simulink model "SF051A_SnsrOffsLrng"  (R2013b)
settings: Solver=FixedStepDiscrete  SolverMode=SingleTasking  StartTime=0.0  StopTime=1  FixedStep=0.002  RelTol=1e-3
values from neighbouring files (symbols this model uses):
  ARCHGLBPRM_10MILLISEC_SEC_F32 = DataDict.Constant    [SF051A_SnsrOffsLrng_DataDict.m]
  ARCHGLBPRM_2MILLISEC_SEC_F32 = DataDict.Constant    [SF051A_SnsrOffsLrng_DataDict.m]
  ARCHGLBPRM_2PI_ULS_F32 = DataDict.Constant    [SF051A_SnsrOffsLrng_DataDict.m]
  ARCHGLBPRM_FLOATZEROTHD_ULS_F32 = DataDict.Constant    [SF051A_SnsrOffsLrng_DataDict.m]
  ARCHGLBPRM_PIOVER180_ULS_F32 = DataDict.Constant    [SF051A_SnsrOffsLrng_DataDict.m]
  CNV100MICROSECTOSEC_SECPERCNT_F32 = DataDict.Constant    [SF051A_SnsrOffsLrng_DataDict.m]
  COVRAMTRXNIT_ULS_F32 = DataDict.Constant    [SF051A_SnsrOffsLrng_DataDict.m]
  HWAGHILIM_HWDEG_F32 = DataDict.Constant    [SF051A_SnsrOffsLrng_DataDict.m]
  HWAUTHYTHD_ULS_F32 = DataDict.Constant    [SF051A_SnsrOffsLrng_DataDict.m]
  HWTQLRNGSTSLRND_CNT_U08 = DataDict.Constant    [SF051A_SnsrOffsLrng_DataDict.m]
  HWTQLRNGSTSNEGOFFS_CNT_U08 = DataDict.Constant    [SF051A_SnsrOffsLrng_DataDict.m]
  HWTQLRNGSTSNOTLRND_CNT_U08 = DataDict.Constant    [SF051A_SnsrOffsLrng_DataDict.m]
  HWTQLRNGSTSPOSOFFS_CNT_U08 = DataDict.Constant    [SF051A_SnsrOffsLrng_DataDict.m]
  HWTQLRNGSTSZEROOFFS_CNT_U08 = DataDict.Constant    [SF051A_SnsrOffsLrng_DataDict.m]
  IDYMTRX_ULS_F32 = DataDict.Constant    [SF051A_SnsrOffsLrng_DataDict.m]
  IVS10MS_ULSPERSEC_F32 = DataDict.Constant    [SF051A_SnsrOffsLrng_DataDict.m]
  LRNGFILTICON_ULS_F32 = DataDict.Constant    [SF051A_SnsrOffsLrng_DataDict.m]
  ONE_ULS_F32 = DataDict.Constant    [SF051A_SnsrOffsLrng_DataDict.m]
  SnsrOffsLrnd = DataDict.NVM    [SF051A_SnsrOffsLrng_DataDict.m]
  SnsrOffsLrngFctEna = DataDict.Calibration    [SF051A_SnsrOffsLrng_DataDict.m]
  SnsrOffsLrngHwAgLrngDrvgDstThd = DataDict.Calibration    [SF051A_SnsrOffsLrng_DataDict.m]
  SnsrOffsLrngHwAgLrngEna = DataDict.Calibration    [SF051A_SnsrOffsLrng_DataDict.m]
  SnsrOffsLrngHwAgLrngHwVelThd = DataDict.Calibration    [SF051A_SnsrOffsLrng_DataDict.m]
  SnsrOffsLrngHwAgLrngSysTqThd = DataDict.Calibration    [SF051A_SnsrOffsLrng_DataDict.m]
  SnsrOffsLrngHwAgLrngSysTqThdMed = DataDict.Calibration    [SF051A_SnsrOffsLrng_DataDict.m]
  SnsrOffsLrngHwAgLrngSysTqThdTrustd = DataDict.Calibration    [SF051A_SnsrOffsLrng_DataDict.m]
  SnsrOffsLrngHwAgLrngSysTqThdWide = DataDict.Calibration    [SF051A_SnsrOffsLrng_DataDict.m]
  SnsrOffsLrngHwAgLrngTi = DataDict.Calibration    [SF051A_SnsrOffsLrng_DataDict.m]
  SnsrOffsLrngHwAgLrngVehSpdThd = DataDict.Calibration    [SF051A_SnsrOffsLrng_DataDict.m]
  SnsrOffsLrngHwAgLrngYawOffsDbnd = DataDict.Calibration    [SF051A_SnsrOffsLrng_DataDict.m]
  SnsrOffsLrngHwAgLrngYawRateThd = DataDict.Calibration    [SF051A_SnsrOffsLrng_DataDict.m]
  SnsrOffsLrngHwAgOffsLim = DataDict.Calibration    [SF051A_SnsrOffsLrng_DataDict.m]
  SnsrOffsLrngHwTqLrngEna = DataDict.Calibration    [SF051A_SnsrOffsLrng_DataDict.m]
  SnsrOffsLrngHwTqLrngEnaTiThd = DataDict.Calibration    [SF051A_SnsrOffsLrng_DataDict.m]
  SnsrOffsLrngHwTqLrngHwAgDbnd = DataDict.Calibration    [SF051A_SnsrOffsLrng_DataDict.m]
  SnsrOffsLrngHwTqLrngHwAgThd = DataDict.Calibration    [SF051A_SnsrOffsLrng_DataDict.m]
  SnsrOffsLrngHwTqLrngHwTqThd = DataDict.Calibration    [SF051A_SnsrOffsLrng_DataDict.m]
  SnsrOffsLrngHwTqLrngHwTqZeroOffsThd = DataDict.Calibration    [SF051A_SnsrOffsLrng_DataDict.m]
  SnsrOffsLrngHwTqLrngHwVelThd = DataDict.Calibration    [SF051A_SnsrOffsLrng_DataDict.m]
  SnsrOffsLrngHwTqLrngMeasTi = DataDict.Calibration    [SF051A_SnsrOffsLrng_DataDict.m]
  SnsrOffsLrngHwTqLrngMeasTiScar = DataDict.Calibration    [SF051A_SnsrOffsLrng_DataDict.m]
  SnsrOffsLrngHwTqLrngSampleImbThd1 = DataDict.Calibration    [SF051A_SnsrOffsLrng_DataDict.m]
  SnsrOffsLrngHwTqLrngSampleImbThd2 = DataDict.Calibration    [SF051A_SnsrOffsLrng_DataDict.m]
  SnsrOffsLrngHwTqLrngSampleThd1 = DataDict.Calibration    [SF051A_SnsrOffsLrng_DataDict.m]
  SnsrOffsLrngHwTqLrngSampleThd2 = DataDict.Calibration    [SF051A_SnsrOffsLrng_DataDict.m]
  SnsrOffsLrngHwTqLrngTiWghtCoeff = DataDict.Calibration    [SF051A_SnsrOffsLrng_DataDict.m]
  SnsrOffsLrngHwTqLrngVehSpdThd = DataDict.Calibration    [SF051A_SnsrOffsLrng_DataDict.m]
  SnsrOffsLrngHwTqOffsLim = DataDict.Calibration    [SF051A_SnsrOffsLrng_DataDict.m]
  SnsrOffsLrngSampleCntForHwTqLrngRst = DataDict.Calibration    [SF051A_SnsrOffsLrng_DataDict.m]
  SnsrOffsLrngTqInpDetnPwrEstimnThd = DataDict.Calibration    [SF051A_SnsrOffsLrng_DataDict.m]
  SnsrOffsLrngTqInpDetnSinGenrAmp = DataDict.Calibration    [SF051A_SnsrOffsLrng_DataDict.m]
  SnsrOffsLrngTqInpDetnSinGenrFrq = DataDict.Calibration    [SF051A_SnsrOffsLrng_DataDict.m]
  SnsrOffsLrngTqInpDetnStg1FilGain = DataDict.Calibration    [SF051A_SnsrOffsLrng_DataDict.m]
  SnsrOffsLrngTqInpDetnStg1WinSize = DataDict.Calibration    [SF051A_SnsrOffsLrng_DataDict.m]
  SnsrOffsLrngTqInpDetnStg2FilGainCen = DataDict.Calibration    [SF051A_SnsrOffsLrng_DataDict.m]
  SnsrOffsLrngTqInpDetnStg2FilGainDwn = DataDict.Calibration    [SF051A_SnsrOffsLrng_DataDict.m]
  SnsrOffsLrngTqInpDetnStg2FilGainUp = DataDict.Calibration    [SF051A_SnsrOffsLrng_DataDict.m]
  SnsrOffsLrngTqInpDetnStg2WinSize = DataDict.Calibration    [SF051A_SnsrOffsLrng_DataDict.m]
  SnsrOffsLrngYawLrngEna = DataDict.Calibration    [SF051A_SnsrOffsLrng_DataDict.m]
  SnsrOffsLrngYawLrngHwAgThd = DataDict.Calibration    [SF051A_SnsrOffsLrng_DataDict.m]
  SnsrOffsLrngYawLrngTi = DataDict.Calibration    [SF051A_SnsrOffsLrng_DataDict.m]
  SnsrOffsLrngYawLrngYawAThd = DataDict.Calibration    [SF051A_SnsrOffsLrng_DataDict.m]
  SnsrOffsLrngYawOffsFrshTiThd = DataDict.Calibration    [SF051A_SnsrOffsLrng_DataDict.m]
  SnsrOffsLrngYawRateOffsLim = DataDict.Calibration    [SF051A_SnsrOffsLrng_DataDict.m]
  SPDCNVN_MTRPERSECPERKPH_F32 = DataDict.Constant    [SF051A_SnsrOffsLrng_DataDict.m]
  SysGlbPrmSysTqRat = DataDict.ImprtdCal    [SF051A_SnsrOffsLrng_DataDict.m]
  TISTEP10MS_MINS_F32 = DataDict.Constant    [SF051A_SnsrOffsLrng_DataDict.m]
  TQINPDETNLOGGAIN_ULS_F32 = DataDict.Constant    [SF051A_SnsrOffsLrng_DataDict.m]
  YAWELPDTIHILIM_MINS_F32 = DataDict.Constant    [SF051A_SnsrOffsLrng_DataDict.m]
  YAWRATENOISE_VEHDEGPERSEC_F32 = DataDict.Constant    [SF051A_SnsrOffsLrng_DataDict.m]
  ZERO_ULS_F32 = DataDict.Constant    [SF051A_SnsrOffsLrng_DataDict.m]
  ZEROVECT_ULS_F32 = DataDict.Constant    [SF051A_SnsrOffsLrng_DataDict.m]
undefined symbols (not defined in the file or in its folder): NvmGetErrSts1
libraries: Fil x34, NxtrLim x20, FixdToFloat x17, FloatToFixd x16, simulink x12, NxtrAbslt x12, NxtrNvM x8, NxtrMath x3
(part 4 of 12)

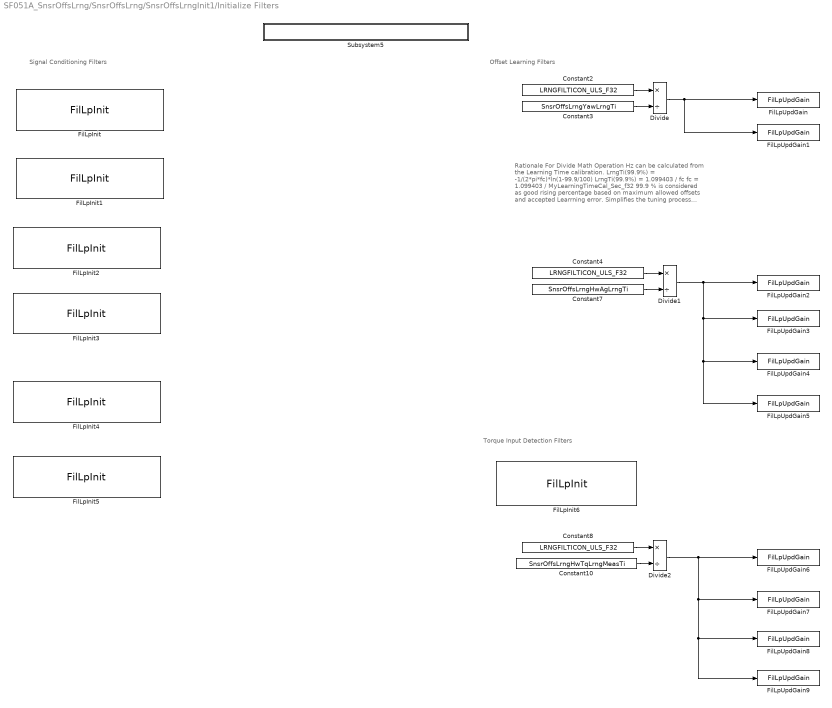
== system SF051A_SnsrOffsLrng/SnsrOffsLrng/SnsrOffsLrngInit1/Initialize Filters ==
  note: Rationale For Divide Math Operation
      |   Hz can be calculated from the Learning Time calibration.
      |   LrngTi(99.9%) = -1/(2*pi*fc)*ln(1-99.9/100)
      |   LrngTi(99.9%) = 1.099403 / fc
      |   fc = 1.099403 / MyLearningTimeCal_Sec_f32
      |
      |   99.9 % is considered as good rising percentage based on
      |   maximum allowed offsets and accepted Learrning error.
      |   Simplifies the tuning process and prevents the customer to
      |   directly find out that we use LPF as the learning method.
  note: Signal Conditioning Filters
  note: Offset Learning Filters
  note: Torque Input Detection Filters
  Constant10 : Constant  Value=SnsrOffsLrngHwTqLrngMeasTi
  Constant2 : Constant  Value=LRNGFILTICON_ULS_F32
  Constant3 : Constant  Value=SnsrOffsLrngYawLrngTi
  Constant4 : Constant  Value=LRNGFILTICON_ULS_F32
  Constant7 : Constant  Value=SnsrOffsLrngHwAgLrngTi
  Constant8 : Constant  Value=LRNGFILTICON_ULS_F32
  Divide : Product  Inputs=*/
  Divide1 : Product  Inputs=*/
  Divide2 : Product  Inputs=*/
  FilLpInit : Fil/FilLpInit  Ic=0  Ts=ARCHGLBPRM_10MILLISEC_SEC_F32  Freq=SnsrOffsLrngYawRateCdngFilFrq  StVar=YawCdngFil1
  FilLpInit1 : Fil/FilLpInit  Ic=0  Ts=ARCHGLBPRM_10MILLISEC_SEC_F32  Freq=SnsrOffsLrngYawRateCdngFilFrq  StVar=YawCdngFil2
  FilLpInit2 : Fil/FilLpInit  Ic=0  Ts=ARCHGLBPRM_10MILLISEC_SEC_F32  Freq=SnsrOffsLrngYawACdngFilFrq  StVar=YawACdngFil
  FilLpInit3 : Fil/FilLpInit  Ic=0  Ts=ARCHGLBPRM_10MILLISEC_SEC_F32  Freq=SnsrOffsLrngTqAndAgFilFrq  StVar=HwAgCdngFil
  FilLpInit4 : Fil/FilLpInit  Ic=0  Ts=ARCHGLBPRM_10MILLISEC_SEC_F32  Freq=SnsrOffsLrngHwVelFilFrq  StVar=HwVelCdngFil
  FilLpInit5 : Fil/FilLpInit  Ic=0  Ts=ARCHGLBPRM_10MILLISEC_SEC_F32  Freq=SnsrOffsLrngTqAndAgFilFrq  StVar=SysTqCdngFil
  FilLpInit6 : Fil/FilLpInit  Ic=0  Ts=ARCHGLBPRM_2MILLISEC_SEC_F32  Freq=SnsrOffsLrngTqInpDetnHwTqFilFrq  StVar=TqInpDetnHwTqFil
  FilLpUpdGain : Fil/FilLpUpdGain  Ts=ARCHGLBPRM_10MILLISEC_SEC_F32  StVar=YawLrngFil1
      settings: AttributesFormatString=|
      | Ts: %<Ts>
      | StVar: %<StVar>
  FilLpUpdGain1 : Fil/FilLpUpdGain  Ts=ARCHGLBPRM_10MILLISEC_SEC_F32  StVar=YawLrngFil2
      settings: AttributesFormatString=|
      | Ts: %<Ts>
      | StVar: %<StVar>
  FilLpUpdGain2 : Fil/FilLpUpdGain  Ts=ARCHGLBPRM_10MILLISEC_SEC_F32  StVar=HwAgLrngFil1
      settings: AttributesFormatString=|
      | Ts: %<Ts>
      | StVar: %<StVar>
  FilLpUpdGain3 : Fil/FilLpUpdGain  Ts=ARCHGLBPRM_10MILLISEC_SEC_F32  StVar=HwAgLrngFil2
      settings: AttributesFormatString=|
      | Ts: %<Ts>
      | StVar: %<StVar>
  FilLpUpdGain4 : Fil/FilLpUpdGain  Ts=ARCHGLBPRM_10MILLISEC_SEC_F32  StVar=HwAgLrngSysTqFil1
      settings: AttributesFormatString=|
      | Ts: %<Ts>
      | StVar: %<StVar>
  FilLpUpdGain5 : Fil/FilLpUpdGain  Ts=ARCHGLBPRM_10MILLISEC_SEC_F32  StVar=HwAgLrngSysTqFil2
      settings: AttributesFormatString=|
      | Ts: %<Ts>
      | StVar: %<StVar>
  FilLpUpdGain6 : Fil/FilLpUpdGain  Ts=ARCHGLBPRM_2MILLISEC_SEC_F32  StVar=HwTqMeasFil1
      settings: AttributesFormatString=|
      | Ts: %<Ts>
      | StVar: %<StVar>
  FilLpUpdGain7 : Fil/FilLpUpdGain  Ts=ARCHGLBPRM_2MILLISEC_SEC_F32  StVar=HwTqMeasFil2
      settings: AttributesFormatString=|
      | Ts: %<Ts>
      | StVar: %<StVar>
  FilLpUpdGain8 : Fil/FilLpUpdGain  Ts=ARCHGLBPRM_2MILLISEC_SEC_F32  StVar=HwAgMeasFil1
      settings: AttributesFormatString=|
      | Ts: %<Ts>
      | StVar: %<StVar>
  FilLpUpdGain9 : Fil/FilLpUpdGain  Ts=ARCHGLBPRM_2MILLISEC_SEC_F32  StVar=HwAgMeasFil2
      settings: AttributesFormatString=|
      | Ts: %<Ts>
      | StVar: %<StVar>
  Subsystem5 : Subsystem  Description=|  mask(Copyright Information){none=on}
      | Copyright info block.                                               
      |                                                                     
      | Place copyright information at the top of every subsystem in design.
      mask prompts: none "No parameters"
      mask help: Place copyright information at the top of every subsystem in design.
      mask Display:
      | NxtrConf = 'Nexteer Confidential';
      | 
      | sys = bdroot; %handle for the current model ("system")
      | first = get_param(sys,'Created');
      | first = first(end-3:end);  %year is last four digits
      | 
      | last = get_param(sys,'LastModifiedDate');
      | if isempty(last)
      |     last = datestr(now,'yyyy');
      | else
      |     last = last(end-3:end);
      | end
      | 
      | if strcmp(first,last)
      |     fprintf('%s -- Copyright %s Nexteer',NxtrConf,first)
      | else
      |     fprintf('%s -- %s%s- %s Nexteer',NxtrConf,char(169),first,last)
      | end
  wires:
  Constant2/1 -> Divide/1
  Constant3/1 -> Divide/2
  Constant4/1 -> Divide1/1
  Constant7/1 -> Divide1/2
  Divide/1 -> FilLpUpdGain1/1, FilLpUpdGain/1
  Constant8/1 -> Divide2/1
  Constant10/1 -> Divide2/2
  Divide2/1 -> FilLpUpdGain9/1, FilLpUpdGain8/1, FilLpUpdGain7/1, FilLpUpdGain6/1
  Divide1/1 -> FilLpUpdGain5/1, FilLpUpdGain4/1, FilLpUpdGain3/1, FilLpUpdGain2/1

== system SF051A_SnsrOffsLrng/SnsrOffsLrng/SnsrOffsLrngInit1/NVM Management ==
  note: This output shall have constant values during the whole ignition cycle.  Learning that occurs in periodic
      |  runnables are applied at the next ignition cycle.
  Constant7 : Constant  RequirementInfo="{'linktype_rmi_doors' '0000babd (/E-STEER Core/SubSystem Specifications/Application Functions/SF051A Sensor Offset Learning)' '#SF051A_45' 'true' 'REQ:  SF051A_45' '' ; 'linktype_rmi_doors' '0000babd (/E-STEER Core/SubSystem Specifications/Application Functions/SF051A Sensor Offset Learning)' '#SF051A_245' 'true' 'REQ:  SF051A_245' '' ; 'linktype_rmi_doors' '0000babd (/E-STEER Core/SubSystem Specifications/Application Functions/SF051A Sensor Offset Learning)' '#SF051A_26' 'true' 'REQ:  SF051A_26' '' ; 'linktype_rmi_doors' '0000babd (/E-STEER Core/SubSystem Specifications/Application Functions/SF051A Sensor Offset Learning)' '#SF051A_244' 'true' 'REQ:  SF051A_244' '' } %GIDa_ef7e5e32_645a_4c45_b476_49e4e533fe27"  Value=SnsrOffsLrngFctEna
  Data Invalid : Subsystem  RequirementInfo="{'linktype_rmi_doors' '0000babd (/E-STEER Core/SubSystem Specifications/Application Functions/SF051A Sensor Offset Learning)' '#SF051A_209' 'true' 'REQ:  SF051A_209' '' ; 'linktype_rmi_doors' '0000babd (/E-STEER Core/SubSystem Specifications/Application Functions/SF051A Sensor Offset Learning)' '#SF051A_81' 'true' 'REQ:  SF051A_81' '' } %GIDa_5e0fb5f6_aa15_4f9e_ae35_640380acf82a"  TreatAsAtomicUnit=on
  Data Valid : Subsystem  RequirementInfo="{'linktype_rmi_doors' '0000babd (/E-STEER Core/SubSystem Specifications/Application Functions/SF051A Sensor Offset Learning)' '#SF051A_46' 'true' 'REQ:  SF051A_46' '' } %GIDa_66d36710_a25b_4f66_be75_e056640be4ef"  TreatAsAtomicUnit=on
  Enumerated Constant : simulink/Sources/Enumerated Constant  RequirementInfo="{'linktype_rmi_doors' '0000babd (/E-STEER Core/SubSystem Specifications/Application Functions/SF051A Sensor Offset Learning)' '#SF051A_209' 'true' 'REQ:  SF051A_209' '' } %GIDa_4ba5cf2e_8700_4b79_8477_f6e2e1d33177"  OutDataTypeStr=Enum: NvmGetErrSts1  Value=NvmGetErrSts1.REQUEST_OK  SampleTime=inf
  HwAgOffs_Merge : Merge  Inputs=3
  HwTqOffs_Merge : Merge  Inputs=3
  If : If  RequirementInfo="{'linktype_rmi_doors' '0000babd (/E-STEER Core/SubSystem Specifications/Application Functions/SF051A Sensor Offset Learning)' '#SF051A_209' 'true' 'REQ:  SF051A_209' '' ; 'linktype_rmi_doors' '0000babd (/E-STEER Core/SubSystem Specifications/Application Functions/SF051A Sensor Offset Learning)' '#SF051A_45' 'true' 'REQ:  SF051A_45' '' ; 'linktype_rmi_doors' '0000babd (/E-STEER Core/SubSystem Specifications/Application Functions/SF051A Sensor Offset Learning)' '#SF051A_245' 'true' 'REQ:  SF051A_245' '' ; 'linktype_rmi_doors' '0000babd (/E-STEER Core/SubSystem Specifications/Application Functions/SF051A Sensor Offset Learning)' '#SF051A_244' 'true' 'REQ:  SF051A_244' '' ; 'linktype_rmi_doors' '0000babd (/E-STEER Core/SubSystem Specifications/Application Functions/SF051A Sensor Offset Learning)' '#SF051A_26' 'true' 'REQ: SF051A_26' '' } %GIDa_d5ac3c33_f41d_4c7c_b2fe_83a09c61ef65"  NumInputs=2  IfExpression=~u1  ElseIfExpressions=u2
  LimStat_f32_1 : NxtrLim/LimStat_f32  LoLim=VehYawRateOffs.EngMin  HiLim=VehYawRateOffs.EngMax
      settings: AttributesFormatString=|
      | Low Limit: %<LoLim>
      | High Limit:%<HiLim>
  LimStat_f32_2 : NxtrLim/LimStat_f32  LoLim=HwAgOffs.EngMin  HiLim=HwAgOffs.EngMax
      settings: AttributesFormatString=|
      | Low Limit: %<LoLim>
      | High Limit:%<HiLim>
  LimStat_f32_3 : NxtrLim/LimStat_f32  LoLim=HwTqOffs.EngMin  HiLim=HwTqOffs.EngMax
      settings: AttributesFormatString=|
      | Low Limit: %<LoLim>
      | High Limit:%<HiLim>
  NVM Quality Check : NxtrNvM/Get Error Status  RequirementInfo="{'linktype_rmi_doors' '0000babd (/E-STEER Core/SubSystem Specifications/Application Functions/SF051A Sensor Offset Learning)' '#SF051A_209' 'true' 'REQ:  SF051A_209' '' } %GIDa_2938958a_fdd5_4115_b739_a05bc2c67ca1"  FuncName=Get Error Status  NvMBlockName=SnsrOffsLrnd  VoidFuncRtn=on  ReqResPtr_DSN=NvMGES_ReqResPtr  Return_DSN=NvMGES_ReqStdReturn
      settings: AttributesFormatString=%<FuncName>
  Not Enabled : Subsystem  RequirementInfo="{'linktype_rmi_doors' '0000babd (/E-STEER Core/SubSystem Specifications/Application Functions/SF051A Sensor Offset Learning)' '#SF051A_45' 'true' 'REQ: SF051A_45' '' ; 'linktype_rmi_doors' '0000babd (/E-STEER Core/SubSystem Specifications/Application Functions/SF051A Sensor Offset Learning)' '#SF051A_245' 'true' 'REQ:  SF051A_245' '' ; 'linktype_rmi_doors' '0000babd (/E-STEER Core/SubSystem Specifications/Application Functions/SF051A Sensor Offset Learning)' '#SF051A_244' 'true' 'REQ:  SF051A_244' '' } %GIDa_33e38bd6_ef28_4946_a942_13c33251a399"  TreatAsAtomicUnit=on
  Relational Operator : RelationalOperator  RequirementInfo="{'linktype_rmi_doors' '0000babd (/E-STEER Core/SubSystem Specifications/Application Functions/SF051A Sensor Offset Learning)' '#SF051A_209' 'true' 'REQ:  SF051A_209' '' } %GIDa_f5be09a0_ba21_4755_8937_69973fb75b04"  Operator=~=  OutDataTypeStr=boolean
  Subsystem5 : Subsystem  Description=|  mask(Copyright Information){none=on}
      | Copyright info block.                                               
      |                                                                     
      | Place copyright information at the top of every subsystem in design.
      mask prompts: none "No parameters"
      mask help: Place copyright information at the top of every subsystem in design.
      mask Display:
      | NxtrConf = 'Nexteer Confidential';
      | 
      | sys = bdroot; %handle for the current model ("system")
      | first = get_param(sys,'Created');
      | first = first(end-3:end);  %year is last four digits
      | 
      | last = get_param(sys,'LastModifiedDate');
      | if isempty(last)
      |     last = datestr(now,'yyyy');
      | else
      |     last = last(end-3:end);
      | end
      | 
      | if strcmp(first,last)
      |     fprintf('%s -- Copyright %s Nexteer',NxtrConf,first)
      | else
      |     fprintf('%s -- %s%s- %s Nexteer',NxtrConf,char(169),first,last)
      | end
  YwRateOffs_Merge : Merge  Inputs=3
  VehYawRateOffs : Outport
  HwAgOffs : Outport  Port=2
  HwTqOffs : Outport  Port=3
  wires:
  NVM Quality Check/1 -> Relational Operator/1
  Enumerated Constant/1 -> Relational Operator/2
  Relational Operator/1 -> If/2
  YwRateOffs_Merge/1 -> LimStat_f32_1/1
  HwAgOffs_Merge/1 -> LimStat_f32_2/1
  HwTqOffs_Merge/1 -> LimStat_f32_3/1
  Constant7/1 -> If/1
  Not Enabled/1(YawOffs) -> YwRateOffs_Merge/1
  Not Enabled/2(HwAgOffs) -> HwAgOffs_Merge/1
  Data Invalid/1(YawOffs) -> YwRateOffs_Merge/2
  Data Valid/1(YawOffs) -> YwRateOffs_Merge/3
  Data Invalid/2(HwAgOffs) -> HwAgOffs_Merge/2
  Data Valid/2(HwAgOffs) -> HwAgOffs_Merge/3
  Not Enabled/3(HwTqOffs) -> HwTqOffs_Merge/1
  Data Valid/3(HwTqOffs) -> HwTqOffs_Merge/3
  Data Invalid/3(HwTqOffs) -> HwTqOffs_Merge/2
  If/1 -> Not Enabled/Action
  If/2 -> Data Invalid/Action
  If/3 -> Data Valid/Action
  LimStat_f32_1/1 -> VehYawRateOffs/1
  LimStat_f32_2/1 -> HwAgOffs/1
  LimStat_f32_3/1 -> HwTqOffs/1

== system SF051A_SnsrOffsLrng/SnsrOffsLrng/SnsrOffsLrngInit1/Subsystem5 ==

== system SF051A_SnsrOffsLrng/SnsrOffsLrng/SnsrOffsLrngPer1/EnableLearning ==
  note: 1 ==  Torque Input is present
      | 0 == Torque Input is NOT present
  note: 1 ==  TID output Valid
      | 0 == TID output Inalid
  note: A Validity flag is needed because
      | TID takes some time to give a valid
      | TorqueInputPresence output.
  VehSpd : Inport
  HwVel : Inport  Port=2
  HwTq : Inport  Port=3
  HwAg : Inport  Port=4
  Action Port : ActionPort  ActionType=then
  Data Store Read : DataStoreRead  Priority=1  DataStoreName=HwTqLrngTqInpDetnEnaPrev
      settings: AttributesFormatString=priority: %<Priority>
  Data Store Write : DataStoreWrite  Priority=2  DataStoreName=HwTqLrngTqInpDetnEnaPrev
      settings: AttributesFormatString=priority: %<Priority>
  Default_TqInpDetn : Subsystem  RequirementInfo="{'linktype_rmi_doors' '0000babd (/E-STEER Core/SubSystem Specifications/Application Functions/SF051A Sensor Offset Learning)' '#SF051A_164' 'true' 'REQ:  SF051A_164' '' } %GIDa_fb449d68_977a_4a81_8991_2af0d6cd2502"  TreatAsAtomicUnit=on
  Display : DataStoreWrite  DataStoreName=dSnsrOffsLrngHwTqLrngTqInpPrsnt
  Display1 : DataStoreWrite  DataStoreName=dSnsrOffsLrngHwTqLrngTqInpPrsntVld
  EnablingConditions : Subsystem
  Eval_Time : Subsystem  RequirementInfo="{'linktype_rmi_doors' '0000babd (/E-STEER Core/SubSystem Specifications/Application Functions/SF051A Sensor Offset Learning)' '#SF051A_164' 'true' 'REQ:  SF051A_164' '' } %GIDa_327f7daf_7ea8_4042_8268_63038c55edb2"  TreatAsAtomicUnit=on
  False_Reset : Subsystem  RequirementInfo="{'linktype_rmi_doors' '0000babd (/E-STEER Core/SubSystem Specifications/Application Functions/SF051A Sensor Offset Learning)' '#SF051A_164' 'true' 'REQ:  SF051A_164' '' } %GIDa_a71081cc_a288_4d1b_bc6a_ea8c5fbdf044"  TreatAsAtomicUnit=on
  Filter_HwTq : Subsystem
  If1 : If  IfExpression=u1
  If2 : If  RequirementInfo="{'linktype_rmi_doors' '0000babd (/E-STEER Core/SubSystem Specifications/Application Functions/SF051A Sensor Offset Learning)' '#SF051A_164' 'true' 'REQ:  SF051A_164' '' } %GIDa_77b22b4b_0372_4138_b51c_8fea69f42076"  NumInputs=2  IfExpression=u1 & ~u2
  MergeEnable : Merge
  Merge_Present : Merge
  Merge_Validity : Merge
  Perform_TqInpDetn : Subsystem  RequirementInfo="{'linktype_rmi_doors' '0000babd (/E-STEER Core/SubSystem Specifications/Application Functions/SF051A Sensor Offset Learning)' '#SF051A_166' 'true' 'REQ:  SF051A_166' '' ; 'linktype_rmi_doors' '0000babd (/E-STEER Core/SubSystem Specifications/Application Functions/SF051A Sensor Offset Learning)' '#SF051A_164' 'true' 'REQ:  SF051A_164' '' } %GIDa_2f938550_6884_4202_ab7e_29e5b30f1426"  TreatAsAtomicUnit=on
  Subsystem5 : Subsystem  Description=|  mask(Copyright Information){none=on}
      | Copyright info block.                                               
      |                                                                     
      | Place copyright information at the top of every subsystem in design.
      mask prompts: none "No parameters"
      mask help: Place copyright information at the top of every subsystem in design.
      mask Display:
      | NxtrConf = 'Nexteer Confidential';
      | 
      | sys = bdroot; %handle for the current model ("system")
      | first = get_param(sys,'Created');
      | first = first(end-3:end);  %year is last four digits
      | 
      | last = get_param(sys,'LastModifiedDate');
      | if isempty(last)
      |     last = datestr(now,'yyyy');
      | else
      |     last = last(end-3:end);
      | end
      | 
      | if strcmp(first,last)
      |     fprintf('%s -- Copyright %s Nexteer',NxtrConf,first)
      | else
      |     fprintf('%s -- %s%s- %s Nexteer',NxtrConf,char(169),first,last)
      | end
  HwTqLrngEna : Outport
  wires:
  Perform_TqInpDetn/2(TqInpPrsnt) -> Merge_Present/1
  MergeEnable/1 -> HwTqLrngEna/1  "HwTqLrngEna"
  Perform_TqInpDetn/1(TqInpPrsntVld) -> Merge_Validity/1
  EnablingConditions/1(TqInpDetnEna) -> Data Store Write/1, If1/1
  VehSpd/1 -> EnablingConditions/3(VehSpd)
  HwTq/1 -> EnablingConditions/1(HwTq), Filter_HwTq/1(HwTq)
  If1/1 -> Perform_TqInpDetn/Action
  HwVel/1 -> EnablingConditions/2(HwVel)
  HwAg/1 -> EnablingConditions/4(HwAg)
  Data Store Read/1 -> Perform_TqInpDetn/2(TqInpDetnEnaPrev)
  Filter_HwTq/1(HwTqFild) -> Perform_TqInpDetn/1(HwTqFild)
  If1/2 -> Default_TqInpDetn/Action
  Merge_Validity/1 -> Display1/1, If2/1
  Merge_Present/1 -> Display/1, If2/2
  Default_TqInpDetn/1(TqInpPresVld) -> Merge_Validity/2
  Default_TqInpDetn/2(TqInpPrsnt) -> Merge_Present/2
  If2/1 -> Eval_Time/Action
  If2/2 -> False_Reset/Action
  Eval_Time/1(HwTqLrngEna) -> MergeEnable/1
  False_Reset/1(HwTqLrngEna) -> MergeEnable/2

== system SF051A_SnsrOffsLrng/SnsrOffsLrng/SnsrOffsLrngPer1/Hold ==
  Action Port : ActionPort  ActionType=else
  Data Store Read : DataStoreRead  DataStoreName=SnsrOffsLrnd  DataStoreElements=SnsrOffsLrnd.HwTqLrngSts
  Subsystem5 : Subsystem  Description=|  mask(Copyright Information){none=on}
      | Copyright info block.                                               
      |                                                                     
      | Place copyright information at the top of every subsystem in design.
      mask prompts: none "No parameters"
      mask help: Place copyright information at the top of every subsystem in design.
      mask Display:
      | NxtrConf = 'Nexteer Confidential';
      | 
      | sys = bdroot; %handle for the current model ("system")
      | first = get_param(sys,'Created');
      | first = first(end-3:end);  %year is last four digits
      | 
      | last = get_param(sys,'LastModifiedDate');
      | if isempty(last)
      |     last = datestr(now,'yyyy');
      | else
      |     last = last(end-3:end);
      | end
      | 
      | if strcmp(first,last)
      |     fprintf('%s -- Copyright %s Nexteer',NxtrConf,first)
      | else
      |     fprintf('%s -- %s%s- %s Nexteer',NxtrConf,char(169),first,last)
      | end
  LrngSts : Outport
  wires:
  Data Store Read/1 -> LrngSts/1

== system SF051A_SnsrOffsLrng/SnsrOffsLrng/SnsrOffsLrngPer1/Learning ==
  HwTqMeasd : Inport  RequirementInfo="{'linktype_rmi_doors' '0000babd (/E-STEER Core/SubSystem Specifications/Application Functions/SF051A Sensor Offset Learning)' '#SF051A_151' 'true' 'REQ:  SF051A_151' '' } %GIDa_6b91f63c_4aaa_4bfa_9376_f983d0ac1d0d"
  HwAgMeasd : Inport  RequirementInfo="{'linktype_rmi_doors' '0000babd (/E-STEER Core/SubSystem Specifications/Application Functions/SF051A Sensor Offset Learning)' '#SF051A_184' 'true' 'REQ:  SF051A_184' '' } %GIDa_17f43060_1b75_4af3_aca4_9856b43acba3"  Port=2
  Action Port : ActionPort  ActionType=then
  CalculateOnCenterTorqueDrift : Subsystem
  Counter : Subsystem
  Do nothing : Subsystem  TreatAsAtomicUnit=on
  ForgettingFactor : Subsystem
  HwPos vs HwTrq Model : Subsystem  RequirementInfo="{'linktype_rmi_doors' '0000babd (/E-STEER Core/SubSystem Specifications/Application Functions/SF051A Sensor Offset Learning)' '#SF051A_183' 'true' 'REQ:  SF051A_183' '' } %GIDa_2c905265_b62f_4977_a42f_8f81585002d6"
  If : If  RequirementInfo="{'linktype_rmi_doors' '0000babd (/E-STEER Core/SubSystem Specifications/Application Functions/SF051A Sensor Offset Learning)' '#SF051A_191' 'true' 'REQ:  SF051A_191' '' } %GIDa_dee2ea89_ef06_473f_9de3_281c9e94243f"  IfExpression=u1
  Recursive Least Square Regression : Subsystem  RequirementInfo="{'linktype_rmi_doors' '0000babd (/E-STEER Core/SubSystem Specifications/Application Functions/SF051A Sensor Offset Learning)' '#SF051A_183' 'true' 'REQ:  SF051A_183' '' ; 'linktype_rmi_doors' '0000babd (/E-STEER Core/SubSystem Specifications/Application Functions/SF051A Sensor Offset Learning)' '#SF051A_176' 'true' 'REQ:  SF051A_176' '' } %GIDa_c4fca419_8056_4810_9f75_4fe93673b14d"
  Subsystem5 : Subsystem  Description=|  mask(Copyright Information){none=on}
      | Copyright info block.                                               
      |                                                                     
      | Place copyright information at the top of every subsystem in design.
      mask prompts: none "No parameters"
      mask help: Place copyright information at the top of every subsystem in design.
      mask Display:
      | NxtrConf = 'Nexteer Confidential';
      | 
      | sys = bdroot; %handle for the current model ("system")
      | first = get_param(sys,'Created');
      | first = first(end-3:end);  %year is last four digits
      | 
      | last = get_param(sys,'LastModifiedDate');
      | if isempty(last)
      |     last = datestr(now,'yyyy');
      | else
      |     last = last(end-3:end);
      | end
      | 
      | if strcmp(first,last)
      |     fprintf('%s -- Copyright %s Nexteer',NxtrConf,first)
      | else
      |     fprintf('%s -- %s%s- %s Nexteer',NxtrConf,char(169),first,last)
      | end
  Update_NvmRam : Subsystem  TreatAsAtomicUnit=on
  ValidityCheck : Subsystem
  LrngSts : Outport  RequirementInfo="{'linktype_rmi_doors' '0000babd (/E-STEER Core/SubSystem Specifications/Application Functions/SF051A Sensor Offset Learning)' '#SF051A_189' 'true' 'REQ:  SF051A_189' '' } %GIDa_cb6e3e0e_5f89_407b_8d55_a3ac40da5062"
  wires:
  HwTqMeasd/1 -> Recursive Least Square Regression/2(HwTqMeasd)
  ValidityCheck/2(EstimnVld) -> If/1
  HwPos vs HwTrq Model/1(XAry) -> Recursive Least Square Regression/1(XAry)
  Recursive Least Square Regression/2(A2) -> CalculateOnCenterTorqueDrift/2(A2)
  Recursive Least Square Regression/1(HwTqOffsEstimd) -> CalculateOnCenterTorqueDrift/1(HwTqOffsEstimd)
  If/1 -> Update_NvmRam/Action
  CalculateOnCenterTorqueDrift/1(HwTqDriftEstimnOnCentr) -> ValidityCheck/4(HwTqDriftEstimnOnCentr), Update_NvmRam/1(HwTqDriftEstimnOnCentr)
  HwAgMeasd/1 -> Counter/1(HwAgMeasd), HwPos vs HwTrq Model/1(HwAgMeasd)
  Counter/2(SampleCntPos) -> ValidityCheck/2(SampleCntPos)
  Counter/3(SampleCntNeg) -> ValidityCheck/3(SampleCntNeg)
  Counter/1(SampleCntTot) -> ForgettingFactor/1(SampleCntTot), ValidityCheck/1(SampleCntTot)
  ValidityCheck/1(LrngSts) -> LrngSts/1
  If/2 -> Do nothing/Action

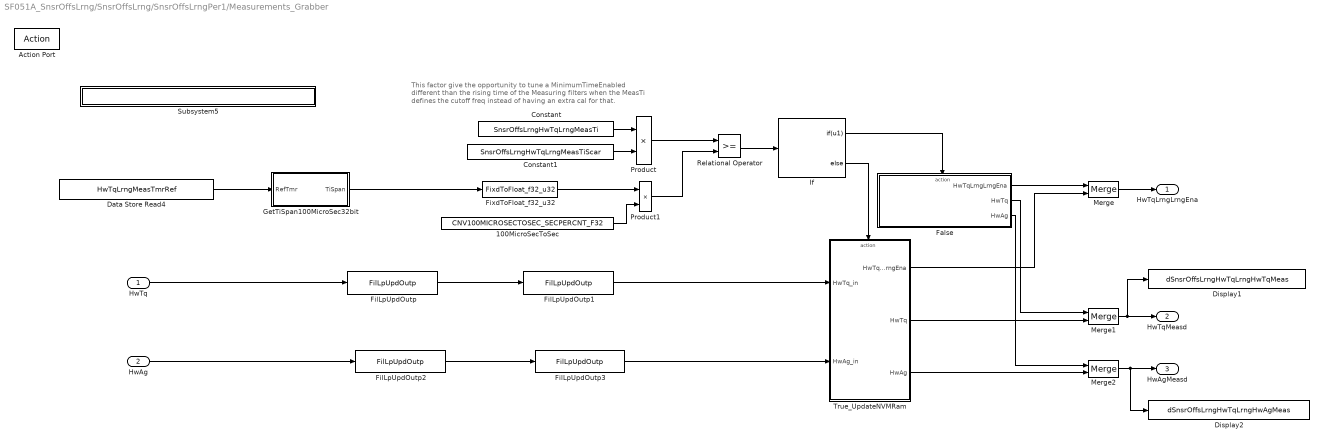
== system SF051A_SnsrOffsLrng/SnsrOffsLrng/SnsrOffsLrngPer1/Measurements_Grabber ==
  note: This factor give the opportunity to tune a MinimumTimeEnabled
      | different than the rising time of the Measuring filters when the
      | MeasTi defines the cutoff freq instead of having an extra cal for that.
  HwTq : Inport
  HwAg : Inport  Port=2
  Action Port : ActionPort  ActionType=then
  100MicroSecToSec : Constant  RequirementInfo="{'linktype_rmi_doors' '0000babd (/E-STEER Core/SubSystem Specifications/Application Functions/SF051A Sensor Offset Learning)' '#SF051A_157' 'true' 'REQ:  SF051A_157' '' } %GIDa_1d6302b6_0890_412f_a859_74bfec20d446"  Value=CNV100MICROSECTOSEC_SECPERCNT_F32
  Constant : Constant  RequirementInfo="{'linktype_rmi_doors' '0000babd (/E-STEER Core/SubSystem Specifications/Application Functions/SF051A Sensor Offset Learning)' '#SF051A_154' 'true' 'REQ:  SF051A_154' '' } %GIDa_56d7af56_202d_46d9_a752_2427b4d5f9ba"  Value=SnsrOffsLrngHwTqLrngMeasTi
  Constant1 : Constant  RequirementInfo="{'linktype_rmi_doors' '0000babd (/E-STEER Core/SubSystem Specifications/Application Functions/SF051A Sensor Offset Learning)' '#SF051A_154' 'true' 'REQ:  SF051A_154' '' } %GIDa_43669e2c_1f40_44c3_9782_3cb4740960cc"  Value=SnsrOffsLrngHwTqLrngMeasTiScar
  Data Store Read4 : DataStoreRead  RequirementInfo="{'linktype_rmi_doors' '0000babd (/E-STEER Core/SubSystem Specifications/Application Functions/SF051A Sensor Offset Learning)' '#SF051A_157' 'true' 'REQ:  SF051A_157' '' } %GIDa_65b5064f_805f_4fdf_83bd_94b1fd8f7a21"  DataStoreName=HwTqLrngMeasTmrRef
  Display1 : DataStoreWrite  DataStoreName=dSnsrOffsLrngHwTqLrngHwTqMeas
  Display2 : DataStoreWrite  DataStoreName=dSnsrOffsLrngHwTqLrngHwAgMeas
  False : Subsystem  TreatAsAtomicUnit=on
  FilLpUpdOutp : Fil/FilLpUpdOutp  RequirementInfo={'linktype_rmi_doors' '0000babd (/E-STEER Core/SubSystem Specifications/Application Functions/SF051A Sensor Offset Learning)' '#SF051A_160' 'true' 'REQ: SF051A_160' '' } %GIDa_26ea5288_ba22_47ce_b770_d988883014c5  StVar=HwTqMeasFil1
      settings: AttributesFormatString=StVar: %<StVar>
  FilLpUpdOutp1 : Fil/FilLpUpdOutp  RequirementInfo={'linktype_rmi_doors' '0000babd (/E-STEER Core/SubSystem Specifications/Application Functions/SF051A Sensor Offset Learning)' '#SF051A_160' 'true' 'REQ: SF051A_160' '' } %GIDa_44139e70_95ec_4501_a5af_33385ed6259d  StVar=HwTqMeasFil2
      settings: AttributesFormatString=StVar: %<StVar>
  FilLpUpdOutp2 : Fil/FilLpUpdOutp  RequirementInfo="{'linktype_rmi_doors' '0000babd (/E-STEER Core/SubSystem Specifications/Application Functions/SF051A Sensor Offset Learning)' '#SF051A_158' 'true' 'REQ:  SF051A_158' '' } %GIDa_9fa9f170_c827_4adc_97b7_7588f08db092"  StVar=HwAgMeasFil1
      settings: AttributesFormatString=StVar: %<StVar>
  FilLpUpdOutp3 : Fil/FilLpUpdOutp  RequirementInfo="{'linktype_rmi_doors' '0000babd (/E-STEER Core/SubSystem Specifications/Application Functions/SF051A Sensor Offset Learning)' '#SF051A_158' 'true' 'REQ:  SF051A_158' '' } %GIDa_ec48da27_f678_4347_b2ae_cf226b9463d3"  StVar=HwAgMeasFil2
      settings: AttributesFormatString=StVar: %<StVar>
  FixdToFloat_f32_u32 : FixdToFloat/FixdToFloat_f32_u32  RequirementInfo="{'linktype_rmi_doors' '0000babd (/E-STEER Core/SubSystem Specifications/Application Functions/SF051A Sensor Offset Learning)' '#SF051A_157' 'true' 'REQ:  SF051A_157' '' } %GIDa_07d2d055_ba54_400f_9dd7_8d7ebf181d28"  Param1=0
  GetTiSpan100MicroSec32bit : Subsystem  RequirementInfo="{'linktype_rmi_doors' '0000babd (/E-STEER Core/SubSystem Specifications/Application Functions/SF051A Sensor Offset Learning)' '#SF051A_157' 'true' 'REQ:  SF051A_157' '' } %GIDa_c4646d3d_186c_42ea_9c38_ce5192734195"
  If : If  RequirementInfo="{'linktype_rmi_doors' '0000babd (/E-STEER Core/SubSystem Specifications/Application Functions/SF051A Sensor Offset Learning)' '#SF051A_154' 'true' 'REQ:  SF051A_154' '' } %GIDa_693a045f_a63e_4bf8_be35_d7424f1cff2a"  IfExpression=u1
  Merge : Merge
  Merge1 : Merge
  Merge2 : Merge
  Product : Product  RequirementInfo="{'linktype_rmi_doors' '0000babd (/E-STEER Core/SubSystem Specifications/Application Functions/SF051A Sensor Offset Learning)' '#SF051A_154' 'true' 'REQ:  SF051A_154' '' } %GIDa_b1573ed4_9e0f_431c_9c9b_2e204b8164c4"
  Product1 : Product  RequirementInfo="{'linktype_rmi_doors' '0000babd (/E-STEER Core/SubSystem Specifications/Application Functions/SF051A Sensor Offset Learning)' '#SF051A_157' 'true' 'REQ:  SF051A_157' '' } %GIDa_5fd770fc_c814_4d2d_87b8_0219da672283"
  Relational Operator : RelationalOperator  RequirementInfo="{'linktype_rmi_doors' '0000babd (/E-STEER Core/SubSystem Specifications/Application Functions/SF051A Sensor Offset Learning)' '#SF051A_154' 'true' 'REQ:  SF051A_154' '' } %GIDa_c774fe4c_9431_45c3_9948_d4b8c33ac912"  OutDataTypeStr=boolean
  Subsystem5 : Subsystem  Description=|  mask(Copyright Information){none=on}
      | Copyright info block.                                               
      |                                                                     
      | Place copyright information at the top of every subsystem in design.
      mask prompts: none "No parameters"
      mask help: Place copyright information at the top of every subsystem in design.
      mask Display:
      | NxtrConf = 'Nexteer Confidential';
      | 
      | sys = bdroot; %handle for the current model ("system")
      | first = get_param(sys,'Created');
      | first = first(end-3:end);  %year is last four digits
      | 
      | last = get_param(sys,'LastModifiedDate');
      | if isempty(last)
      |     last = datestr(now,'yyyy');
      | else
      |     last = last(end-3:end);
      | end
      | 
      | if strcmp(first,last)
      |     fprintf('%s -- Copyright %s Nexteer',NxtrConf,first)
      | else
      |     fprintf('%s -- %s%s- %s Nexteer',NxtrConf,char(169),first,last)
      | end
  True_UpdateNVMRam : Subsystem  RequirementInfo="{'linktype_rmi_doors' '0000babd (/E-STEER Core/SubSystem Specifications/Application Functions/SF051A Sensor Offset Learning)' '#SF051A_154' 'true' 'REQ:  SF051A_154' '' } %GIDa_d48ccb0c_14d9_44ef_afca_af355b2b18b3"  TreatAsAtomicUnit=on
  HwTqLrngLrngEna : Outport  RequirementInfo={'linktype_rmi_doors' '0000babd (/E-STEER Core/SubSystem Specifications/Application Functions/SF051A Sensor Offset Learning)' '#SF051A_155' 'true' 'REQ: SF051A_155' '' } %GIDa_0258301b_97f1_4648_b177_806518a77288
  " HwTqMeasd" : Outport  RequirementInfo={'linktype_rmi_doors' '0000babd (/E-STEER Core/SubSystem Specifications/Application Functions/SF051A Sensor Offset Learning)' '#SF051A_161' 'true' 'REQ: SF051A_161' '' } %GIDa_0759fd65_0303_4afb_ab27_fdabf4d4d475  Port=2
  HwAgMeasd : Outport  RequirementInfo="{'linktype_rmi_doors' '0000babd (/E-STEER Core/SubSystem Specifications/Application Functions/SF051A Sensor Offset Learning)' '#SF051A_159' 'true' 'REQ:  SF051A_159' '' } %GIDa_3aeccdfb_dedb_4dab_93dd_0c1976115233"  Port=3
  wires:
  Constant/1 -> Product/1
  HwTq/1 -> FilLpUpdOutp/1
  HwAg/1 -> FilLpUpdOutp2/1
  Constant1/1 -> Product/2
  Merge/1 -> HwTqLrngLrngEna/1
  False/1(HwTqLrngLrngEna) -> Merge/1
  If/1 -> False/Action
  If/2 -> True_UpdateNVMRam/Action
  True_UpdateNVMRam/1(HwTqLrngLrngEna) -> Merge/2
  Data Store Read4/1 -> GetTiSpan100MicroSec32bit/1(RefTmr)
  Merge1/1 -> Display1/1, " HwTqMeasd"/1
  Merge2/1 -> Display2/1, HwAgMeasd/1
  FixdToFloat_f32_u32/1 -> Product1/1
  False/2(HwTq) -> Merge1/1
  True_UpdateNVMRam/2(HwTq) -> Merge1/2
  False/3(HwAg) -> Merge2/1
  True_UpdateNVMRam/3(HwAg) -> Merge2/2
  100MicroSecToSec/1 -> Product1/2
  FilLpUpdOutp/1 -> FilLpUpdOutp1/1
  FilLpUpdOutp1/1 -> True_UpdateNVMRam/1(HwTq_in)
  FilLpUpdOutp3/1 -> True_UpdateNVMRam/2(HwAg_in)
  FilLpUpdOutp2/1 -> FilLpUpdOutp3/1
  Product/1 -> Relational Operator/1
  Relational Operator/1 -> If/1
  Product1/1 -> Relational Operator/2
  GetTiSpan100MicroSec32bit/1(TiSpan) -> FixdToFloat_f32_u32/1

== system SF051A_SnsrOffsLrng/SnsrOffsLrng/SnsrOffsLrngPer1/SetFalse ==
  Action Port : ActionPort  ActionType=else
  Constant : Constant  Value=false  OutDataTypeStr=boolean
      settings: AttributesFormatString=%<OutDataTypeStr>
  Subsystem1 : Subsystem  Description=|  mask(Copyright Information){none=on}
      | Copyright info block.                                               
      |                                                                     
      | Place copyright information at the top of every subsystem in design.
      mask prompts: none "No parameters"
      mask help: Place copyright information at the top of every subsystem in design.
      mask Display:
      | NxtrConf = 'Nexteer Confidential';
      | 
      | sys = bdroot; %handle for the current model ("system")
      | first = get_param(sys,'Created');
      | first = first(end-3:end);  %year is last four digits
      | 
      | last = get_param(sys,'LastModifiedDate');
      | if isempty(last)
      |     last = datestr(now,'yyyy');
      | else
      |     last = last(end-3:end);
      | end
      | 
      | if strcmp(first,last)
      |     fprintf('%s -- Copyright %s Nexteer',NxtrConf,first)
      | else
      |     fprintf('%s -- %s%s- %s Nexteer',NxtrConf,char(169),first,last)
      | end
  HwTqLrngEna : Outport
  wires:
  Constant/1 -> HwTqLrngEna/1  "HwTqLrngEna_Cnt_T_lgc"

== system SF051A_SnsrOffsLrng/SnsrOffsLrng/SnsrOffsLrngPer1/Subsystem5 ==

== system SF051A_SnsrOffsLrng/SnsrOffsLrng/SnsrOffsLrngPer1/Zero_GrabberTimer ==
  note: Get Reference Time
  Action Port : ActionPort  ActionType=else
  Constant : Constant  Value=false  OutDataTypeStr=boolean
      settings: AttributesFormatString=%<OutDataTypeStr>
  Data Store Write : DataStoreWrite  RequirementInfo="{'linktype_rmi_doors' '0000babd (/E-STEER Core/SubSystem Specifications/Application Functions/SF051A Sensor Offset Learning)' '#SF051A_156' 'true' 'REQ:  SF051A_156' '' } %GIDa_97664fce_b009_4c7e_a14d_7a7fb17f3fd6"  DataStoreName=HwTqLrngMeasTmrRef
  GetRefTmr100MicroSec32bit : Subsystem  RequirementInfo="{'linktype_rmi_doors' '0000babd (/E-STEER Core/SubSystem Specifications/Application Functions/SF051A Sensor Offset Learning)' '#SF051A_156' 'true' 'REQ:  SF051A_156' '' } %GIDa_7e24fd7a_c205_4536_aae5_5f884d137ede"
  Subsystem5 : Subsystem  Description=|  mask(Copyright Information){none=on}
      | Copyright info block.                                               
      |                                                                     
      | Place copyright information at the top of every subsystem in design.
      mask prompts: none "No parameters"
      mask help: Place copyright information at the top of every subsystem in design.
      mask Display:
      | NxtrConf = 'Nexteer Confidential';
      | 
      | sys = bdroot; %handle for the current model ("system")
      | first = get_param(sys,'Created');
      | first = first(end-3:end);  %year is last four digits
      | 
      | last = get_param(sys,'LastModifiedDate');
      | if isempty(last)
      |     last = datestr(now,'yyyy');
      | else
      |     last = last(end-3:end);
      | end
      | 
      | if strcmp(first,last)
      |     fprintf('%s -- Copyright %s Nexteer',NxtrConf,first)
      | else
      |     fprintf('%s -- %s%s- %s Nexteer',NxtrConf,char(169),first,last)
      | end
  HwTqLrngLrngEna : Outport
  wires:
  GetRefTmr100MicroSec32bit/1(RefTmr) -> Data Store Write/1
  Constant/1 -> HwTqLrngLrngEna/1

== system SF051A_SnsrOffsLrng/SnsrOffsLrng/SnsrOffsLrngPer2/Do nothing ==
  Action Port : ActionPort  ActionType=else
  Subsystem5 : Subsystem  Description=|  mask(Copyright Information){none=on}
      | Copyright info block.                                               
      |                                                                     
      | Place copyright information at the top of every subsystem in design.
      mask prompts: none "No parameters"
      mask help: Place copyright information at the top of every subsystem in design.
      mask Display:
      | NxtrConf = 'Nexteer Confidential';
      | 
      | sys = bdroot; %handle for the current model ("system")
      | first = get_param(sys,'Created');
      | first = first(end-3:end);  %year is last four digits
      | 
      | last = get_param(sys,'LastModifiedDate');
      | if isempty(last)
      |     last = datestr(now,'yyyy');
      | else
      |     last = last(end-3:end);
      | end
      | 
      | if strcmp(first,last)
      |     fprintf('%s -- Copyright %s Nexteer',NxtrConf,first)
      | else
      |     fprintf('%s -- %s%s- %s Nexteer',NxtrConf,char(169),first,last)
      | end

== system SF051A_SnsrOffsLrng/SnsrOffsLrng/SnsrOffsLrngPer2/Enable_Function ==
  note: YOC
  note: POC
  VehSpd : Inport
  HwAg : Inport  Port=2
  VehYawRate : Inport  Port=3
  HwVel : Inport  Port=4
  HwTq : Inport  Port=5
  MotTqCmdCrf : Inport  Port=6
  VehYawRateVld : Inport  Port=7
  HwAgAuthy : Inport  Port=8
  VehSpedVld : Inport  Port=9
  HwTqLrngSts : Inport  Port=10
  Action Port : ActionPort  ActionType=then
  Condition Signals : Subsystem
  Data Store Read : DataStoreRead  DataStoreName=VehYawRateOffsFrsh
  POC : Subsystem  RequirementInfo={'linktype_rmi_doors' '0000babd (/E-STEER Core/SubSystem Specifications/Application Functions/SF051A Sensor Offset Learning)' '#SF051A_60' 'true' 'REQ: SF051A_60' '' } %GIDa_5c0e2b77_ae00_47d4_8e26_40446ee9ed26
  SOaC_HierarchyManager : Subsystem  RequirementInfo="{'linktype_rmi_doors' '0000babd (/E-STEER Core/SubSystem Specifications/Application Functions/SF051A Sensor Offset Learning)' '#SF051A_86' 'true' 'REQ:  SF051A_86' '' } %GIDa_b4a262f8_fff6_4184_b01a_dd0e4f5849be"
  Subsystem5 : Subsystem  Description=|  mask(Copyright Information){none=on}
      | Copyright info block.                                               
      |                                                                     
      | Place copyright information at the top of every subsystem in design.
      mask prompts: none "No parameters"
      mask help: Place copyright information at the top of every subsystem in design.
      mask Display:
      | NxtrConf = 'Nexteer Confidential';
      | 
      | sys = bdroot; %handle for the current model ("system")
      | first = get_param(sys,'Created');
      | first = first(end-3:end);  %year is last four digits
      | 
      | last = get_param(sys,'LastModifiedDate');
      | if isempty(last)
      |     last = datestr(now,'yyyy');
      | else
      |     last = last(end-3:end);
      | end
      | 
      | if strcmp(first,last)
      |     fprintf('%s -- Copyright %s Nexteer',NxtrConf,first)
      | else
      |     fprintf('%s -- %s%s- %s Nexteer',NxtrConf,char(169),first,last)
      | end
  YOC : Subsystem  RequirementInfo="{'linktype_rmi_doors' '0000babd (/E-STEER Core/SubSystem Specifications/Application Functions/SF051A Sensor Offset Learning)' '#SF051A_31' 'true' 'REQ:  SF051A_31' '' ; 'linktype_rmi_doors' '0000babd (/E-STEER Core/SubSystem Specifications/Application Functions/SF051A Sensor Offset Learning)' '#SF051A_98' 'true' 'REQ:  SF051A_98' '' } %GIDa_13d13176_ff4f_4f40_b7d3_67b9eccf2376"
  wires:
  Condition Signals/1(YawRateFild) -> YOC/2(YawRateFild)
  SOaC_HierarchyManager/2(HwAgLrngEna) -> POC/5(HwAgLrngEna)
  SOaC_HierarchyManager/1(YawRateLrngEna) -> [YawRateLrngEna]
  [YawRateLrngEna] -> YOC/1(YawRateLrngEna)
  HwAgAuthy/1 -> SOaC_HierarchyManager/2(HwAgAuthy)
  VehSpedVld/1 -> SOaC_HierarchyManager/3(VehSpdVld)
  VehYawRateVld/1 -> SOaC_HierarchyManager/4(VehYawRateVld)
  VehYawRate/1 -> Condition Signals/1(VehYawRate)
  Condition Signals/5(HwAgFild) -> POC/3(HwAgFild)
  [VehSpd] -> POC/6(VehSpd)
  Condition Signals/3(YawRateCorrd) -> POC/1(YawRateCorrd)
  Condition Signals/6(HwVelFild) -> POC/4(HwVelFild)
  Condition Signals/4(SysTqFild) -> POC/2(SysTqFild)
  HwTqLrngSts/1 -> POC/7(HwTqLrngSts)
  HwTq/1 -> Condition Signals/2(HwTq)
  MotTqCmdCrf/1 -> Condition Signals/3(MotTqCmdCrf)
  HwVel/1 -> Condition Signals/4(HwVel)
  SOaC_HierarchyManager/3(HwAgLrngRst) -> POC/8(HwAgLrngRst)
  Condition Signals/2(YawA) -> YOC/3(YawA)
  HwAg/1 -> [HwAg], Condition Signals/5(HwAg)
  [HwAg] -> YOC/5(HwAg)
  VehSpd/1 -> YOC/4(VehSpd), [VehSpd]
  Data Store Read/1 -> SOaC_HierarchyManager/1(YawRateOffsFrsh)

== system SF051A_SnsrOffsLrng/SnsrOffsLrng/SnsrOffsLrngPer2/Subsystem5 ==

== system SF051A_SnsrOffsLrng/SnsrOffsLrng/RstHwTq/GetRefTmr100MicroSec32bit/CopyRight2 ==

== system SF051A_SnsrOffsLrng/SnsrOffsLrng/SetHwAgOffs/Do nothing/Subsystem5 ==

== system SF051A_SnsrOffsLrng/SnsrOffsLrng/SetHwAgOffs/Reset Learning/Subsystem5 ==

== system SF051A_SnsrOffsLrng/SnsrOffsLrng/SetHwTqOffs/Do nothing/Subsystem5 ==

== system SF051A_SnsrOffsLrng/SnsrOffsLrng/SetHwTqOffs/Reset Learning/GetRefTmr100MicroSec32bit ==
  note: 1 count = 100 uSec
  note: seconds
  note: microseconds
  note: counts
  note: Wrap-to-zero
  note: GetRefTmr100MicroSec32bit
  note: Created Aug 18, 2015
      | Modified Oct 21, 2015
      | Modified Oct 30, 2015
      | Kevin Derry
  CopyRight2 : Subsystem  Description=|  mask(Copyright Information){none=on}
      | Copyright info block.                                               
      |                                                                     
      | Place copyright information at the top of every subsystem in design.
      mask prompts: none "No parameters"
      mask help: Place copyright information at the top of every subsystem in design.
      mask Display:
      | NxtrConf = 'Nexteer Confidential';
      | 
      | sys = bdroot; %handle for the current model ("system")
      | first = get_param(sys,'Created');
      | if(isempty(first))
      |     first = datestr(now,'yyyy');
      | else
      |     first = first(end-3:end);  %year is last four digits
      | end
      | 
      | last = get_param(sys,'LastModifiedDate');
      | if isempty(last)
      |     last = datestr(now,'yyyy');
      | else
      |     last = last(end-3:end);
      | end
      | 
      | if strcmp(first,last)
      |     fprintf('%s -- Copyright %s Nexteer',NxtrConf,first)
      | else
      |     fprintf('%s -- %s%s- %s Nexteer',NxtrConf,char(169),first,last)
      | end
  Count per uSec : Constant  Value=0.01
  Data Store Read1 : DataStoreRead  DataStoreName=SimnTi
  Data Type Conversion1 : DataTypeConversion  OutDataTypeStr=uint32
  Divide1 : Product  Inputs=**
  Divide2 : Product  Inputs=*/
  Max Counts : Constant  Value=2^32-1
  Product1 : Product
  Product2 : Product
  Rounding : Rounding
  Subtract1 : Sum  Inputs=+-
  uSec per Sec : Constant  Value=1000000
  RefTmr : Outport
  wires:
  Product2/1 -> Subtract1/2
  Subtract1/1 -> Data Type Conversion1/1
  Rounding/1 -> Product2/1
  Divide2/1 -> Rounding/1
  Max Counts/1 -> Divide2/2, Product2/2
  Divide1/1 -> Divide2/1, Subtract1/1
  Product1/1 -> Divide1/1
  Count per uSec/1 -> Divide1/2
  uSec per Sec/1 -> Product1/2
  Data Type Conversion1/1 -> RefTmr/1
  Data Store Read1/1 -> Product1/1

== system SF051A_SnsrOffsLrng/SnsrOffsLrng/SetHwTqOffs/Reset Learning/Subsystem5 ==

== system SF051A_SnsrOffsLrng/SnsrOffsLrng/SetYawRateOffs/Do nothing/Subsystem5 ==

== system SF051A_SnsrOffsLrng/SnsrOffsLrng/SetYawRateOffs/Reset Learning/Subsystem5 ==

== system SF051A_SnsrOffsLrng/SnsrOffsLrng/SnsrOffsLrngInit1/Initialize Filters/Subsystem5 ==
